simulink model "zajem_RTDE"  (R2019b)
settings: Solver=FixedStepDiscrete  StartTime=0.0  StopTime=inf  FixedStep=1/500  RelTol=1e-3
libraries: etargetslib x4, dspnetwork x1
settings Model: EnablePacing=on  Creator=ur5e  LastModifiedBy=ur5e

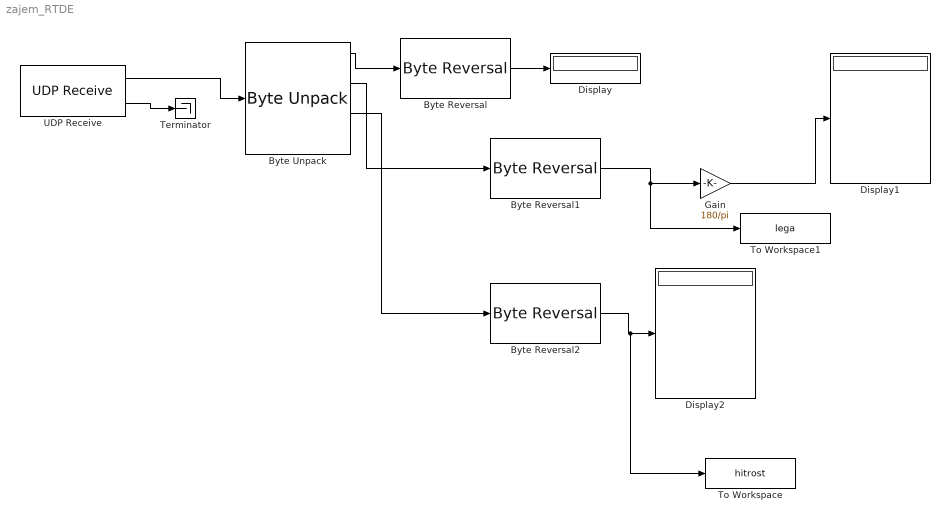
== system zajem_RTDE ==
  Byte Reversal : etargetslib/Byte Reversal  numInp=1
      settings: SourceProductName=MATLAB Coder  SourceProductBaseCode=ME
  Byte Reversal1 : etargetslib/Byte Reversal  numInp=1
      settings: SourceProductName=MATLAB Coder  SourceProductBaseCode=ME
  Byte Reversal2 : etargetslib/Byte Reversal  numInp=1
      settings: SourceProductName=MATLAB Coder  SourceProductBaseCode=ME
  Byte Unpack : etargetslib/Byte Unpack  dimensions={[1], [6],[6],[6]}  datatypes={'double', 'double','double','double'}  byteAlign=1
      settings: SourceProductName=MATLAB Coder
  Display : Display
  Display1 : Display
  Display2 : Display
  Gain : Gain  Gain=180/pi
  Terminator : Terminator
  To Workspace : ToWorkspace  VariableName=hitrost  SaveFormat=Timeseries  SampleTime=-1
  To Workspace1 : ToWorkspace  VariableName=lega  SaveFormat=Timeseries  SampleTime=-1
  UDP Receive : dspnetwork/UDP Receive  localURL='0.0.0.0'  localPort=21000  remoteURL='0.0.0.0'  remotePort=-1  recvBufferSize=8192  dims=152  signalDatatype=uint8  isComplex=off  isVarSize=off  showBlockingTime=off  blockingTime=0  sampletime=1/500  blockPlatform=[]
      settings: SourceProductName=Simulink
  wires:
  UDP Receive/1 -> Byte Unpack/1
  Byte Unpack/2 -> Byte Reversal1/1
  Byte Unpack/1 -> Byte Reversal/1
  UDP Receive/2 -> Terminator/1
  Byte Reversal/1 -> Display/1
  Byte Reversal1/1 -> To Workspace1/1, Gain/1
  Byte Unpack/3 -> Byte Reversal2/1
  Byte Reversal2/1 -> To Workspace/1, Display2/1
  Gain/1 -> Display1/1
